simulink model "softloop1"  (Simulink 3.00)
settings: Solver=ode45  SolverMode=SingleTasking  StartTime=0.0  StopTime=25  MaxStep=.010  RelTol=1e-3  AbsTol=1e-3
settings Model: TimeSaveName=t  SaveOutput=off

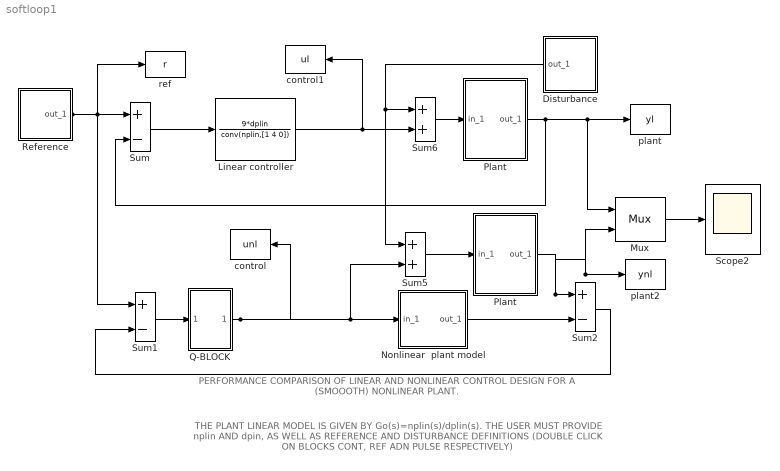
== system softloop1 ==
  note: THE PLANT LINEAR MODEL IS GIVEN BY Go(s)=nplin(s)/dplin(s).
      | THE USER MUST PROVIDE nplin AND dpin, AS WELL AS REFERENCE AND DISTURBANCE DEFINITIONS
      |  (DOUBLE CLICK ON BLOCKS CONT, REF ADN PULSE RESPECTIVELY)
  note: PERFORMANCE COMPARISON OF LINEAR AND NONLINEAR CONTROL DESIGN  FOR A
      | (SMOOOTH) NONLINEAR PLANT.
  Disturbance : Subsystem  Orientation=left  mask(Pulse disturbance){@1=0, @2=5, @3=10}
      mask prompts: @1 "pulse amplitude:"; @2 "initial time:"; @3 "pulse duration:"
      mask help: Pulse
      mask init:
      | D=@1;ti=@2;dt=@3;
      mask Help: This block generates a (one shot) pulse
      mask Display: disp('PULSE')
  Linear controller : TransferFcn  Numerator=9*dplin  Denominator=conv(nplin,[1 4 0])  mask(Controller){@1=1.13, @2=[1 3 1.55]}
      mask prompts: @1 "plant model numerator nplin:"; @2 "plant model denominator dplin:"
      mask help: Plant linear model
      mask init:
      | nplin=@1;dplin=@2;
      mask Display: disp('CONT')
  Mux : Mux  Inputs=2
      settings: DisplayOption=none
  "Nonlinear  plant model " : Subsystem
      mask Type: N.L.Model
      mask Display: disp('N.L.Mod')
  Plant : Subsystem
      mask Type: Plant
      mask Display: disp('Plant');
  "Plant " : Subsystem
      mask Type: Plant
      mask Display: disp('Plant')
  Q-BLOCK : Subsystem
  Reference : Subsystem  mask(Reference){@1=2, @2=0.3, @3=1}
      mask prompts: @1 "mean value Ro:"; @2 "square wave frequency   fsw  [rad/s]:"; @3 "amplitude square wave  asw:"
      mask help: Reference
      mask init:
      | Ro=@1;fsw=@2;asw=@3;
      mask Help: This block generates  a square wave with a user defined mean value.
      mask Display: disp('REF')
  Scope2 : Scope
      settings: TickLabels=on  TimeRange=25.000000  YMin=-4  YMax=4  SaveToWorkspace=off  SaveName=ScopeData  DataFormat=Matrix
  Sum : Sum  Inputs=+-  SaturateOnIntegerOverflow=on
  Sum1 : Sum  Inputs=+-  SaturateOnIntegerOverflow=on
  Sum2 : Sum  Inputs=+-  SaturateOnIntegerOverflow=on
  Sum5 : Sum  Inputs=++  SaturateOnIntegerOverflow=on
  Sum6 : Sum  Inputs=++  SaturateOnIntegerOverflow=on
  control : ToWorkspace  VariableName=unl  SampleTime=0  SaveFormat=Matrix
      settings: Buffer=10000
  control1 : ToWorkspace  VariableName=ul  SampleTime=0  SaveFormat=Matrix
      settings: Buffer=10000
  plant : ToWorkspace  VariableName=yl  SampleTime=0  SaveFormat=Matrix
      settings: Buffer=20000
  plant2 : ToWorkspace  VariableName=ynl  SampleTime=0  SaveFormat=Matrix
      settings: Buffer=20000
  ref : ToWorkspace  VariableName=r  SampleTime=0  SaveFormat=Matrix
      settings: Buffer=20000
  wires:
  Sum/1 -> Linear controller/1
  Plant/1(out_1) -> Sum/2, plant/1, Mux/1
  "Nonlinear  plant model "/1(out_1) -> Sum2/2
  Sum1/1 -> Q-BLOCK/1(in_1)
  Sum2/1 -> Sum1/2
  Q-BLOCK/1(out_1) -> control/1, "Nonlinear  plant model "/1(in_1), Sum5/2
  Sum5/1 -> "Plant "/1(in_1)
  "Plant "/1(out_1) -> Sum2/1, plant2/1, Mux/2
  Mux/1 -> Scope2/1
  Reference/1(out_1) -> Sum/1, Sum1/1, ref/1
  Sum6/1 -> Plant/1(in_1)
  Disturbance/1(out_1) -> Sum6/1, Sum5/1
  Linear controller/1 -> Sum6/2, control1/1

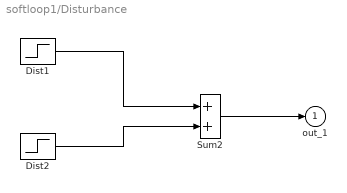
== system softloop1/Disturbance ==
  Dist1 : Step  Time=ti  Before=0  After=D  SampleTime=0
  Dist2 : Step  Time=ti+dt  Before=0  After=-D  SampleTime=0
  Sum2 : Sum  Inputs=++  SaturateOnIntegerOverflow=on
  out_1 : Outport  Port=1  InitialOutput=0
  wires:
  Sum2/1 -> out_1/1
  Dist1/1 -> Sum2/1
  Dist2/1 -> Sum2/2

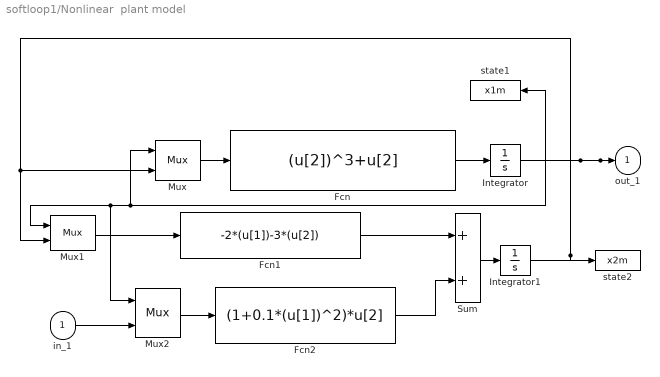
== system softloop1/Nonlinear  plant model  ==
  in_1 : Inport  Port=1  PortWidth=-1  SampleTime=-1  DataType=auto
      settings: SignalType=auto
  Fcn : Fcn  Expr=(u[2])^3+u[2]
  Fcn1 : Fcn  Expr=-2*(u[1])-3*(u[2])
  Fcn2 : Fcn  Expr=(1+0.1*(u[1])^2)*u[2]
  Integrator : Integrator  ExternalReset=none  InitialConditionSource=internal  InitialCondition=0  LimitOutput=off  UpperSaturationLimit=inf  LowerSaturationLimit=-inf  ShowSaturationPort=off  ShowStatePort=off  AbsoluteTolerance=auto
  Integrator1 : Integrator  ExternalReset=none  InitialConditionSource=internal  InitialCondition=0  LimitOutput=off  UpperSaturationLimit=inf  LowerSaturationLimit=-inf  ShowSaturationPort=off  ShowStatePort=off  AbsoluteTolerance=auto
  Mux : Mux  Inputs=2
      settings: DisplayOption=none
  Mux1 : Mux  Inputs=2
      settings: DisplayOption=none
  Mux2 : Mux  Inputs=2
      settings: DisplayOption=none
  Sum : Sum  Inputs=++  SaturateOnIntegerOverflow=on
  state1 : ToWorkspace  VariableName=x1m  SampleTime=0  SaveFormat=Matrix
      settings: Buffer=10000
  state2 : ToWorkspace  VariableName=x2m  SampleTime=0  SaveFormat=Matrix
      settings: Buffer=10000
  out_1 : Outport  Port=1  InitialOutput=0
  wires:
  in_1/1 -> Mux2/2
  Mux/1 -> Fcn/1
  Fcn/1 -> Integrator/1
  Mux1/1 -> Fcn1/1
  Fcn1/1 -> Sum/1
  Sum/1 -> Integrator1/1
  Fcn2/1 -> Sum/2
  Mux2/1 -> Fcn2/1
  Integrator/1 -> out_1/1, Mux/1, Mux1/1, Mux2/1, state1/1
  Integrator1/1 -> Mux1/2, Mux/2, state2/1

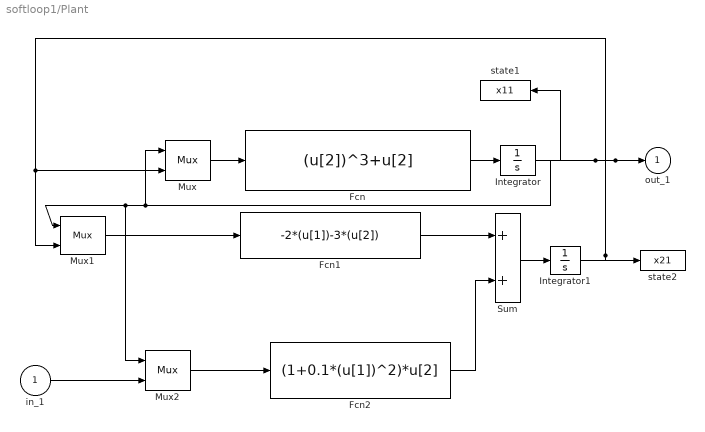
== system softloop1/Plant ==
  in_1 : Inport  Port=1  PortWidth=-1  SampleTime=-1  DataType=auto
      settings: SignalType=auto
  Fcn : Fcn  Expr=(u[2])^3+u[2]
  Fcn1 : Fcn  Expr=-2*(u[1])-3*(u[2])
  Fcn2 : Fcn  Expr=(1+0.1*(u[1])^2)*u[2]
  Integrator : Integrator  ExternalReset=none  InitialConditionSource=internal  InitialCondition=0  LimitOutput=off  UpperSaturationLimit=inf  LowerSaturationLimit=-inf  ShowSaturationPort=off  ShowStatePort=off  AbsoluteTolerance=auto
  Integrator1 : Integrator  ExternalReset=none  InitialConditionSource=internal  InitialCondition=0  LimitOutput=off  UpperSaturationLimit=inf  LowerSaturationLimit=-inf  ShowSaturationPort=off  ShowStatePort=off  AbsoluteTolerance=auto
  Mux : Mux  Inputs=2
      settings: DisplayOption=none
  Mux1 : Mux  Inputs=2
      settings: DisplayOption=none
  Mux2 : Mux  Inputs=2
      settings: DisplayOption=none
  Sum : Sum  Inputs=++  SaturateOnIntegerOverflow=on
  state1 : ToWorkspace  VariableName=x11  SampleTime=0  SaveFormat=Matrix
      settings: Buffer=10000
  state2 : ToWorkspace  VariableName=x21  SampleTime=0  SaveFormat=Matrix
      settings: Buffer=10000
  out_1 : Outport  Port=1  InitialOutput=0
  wires:
  in_1/1 -> Mux2/2
  Mux/1 -> Fcn/1
  Fcn/1 -> Integrator/1
  Mux1/1 -> Fcn1/1
  Fcn1/1 -> Sum/1
  Sum/1 -> Integrator1/1
  Fcn2/1 -> Sum/2
  Mux2/1 -> Fcn2/1
  Integrator/1 -> out_1/1, Mux/1, Mux1/1, Mux2/1, state1/1
  Integrator1/1 -> Mux1/2, Mux/2, state2/1

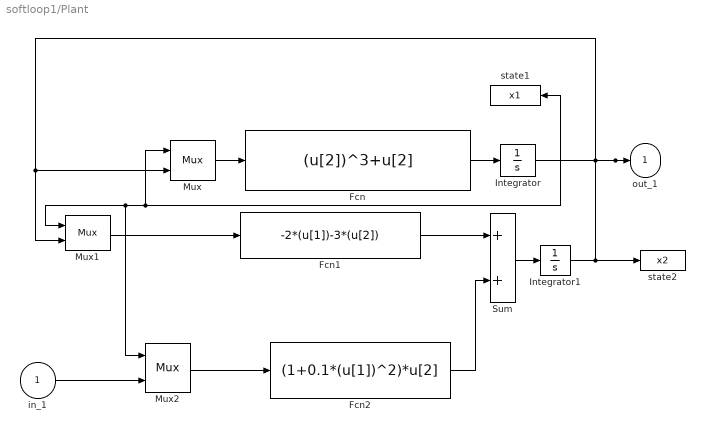
== system softloop1/Plant  ==
  in_1 : Inport  Port=1  PortWidth=-1  SampleTime=-1  DataType=auto
      settings: SignalType=auto
  Fcn : Fcn  Expr=(u[2])^3+u[2]
  Fcn1 : Fcn  Expr=-2*(u[1])-3*(u[2])
  Fcn2 : Fcn  Expr=(1+0.1*(u[1])^2)*u[2]
  Integrator : Integrator  ExternalReset=none  InitialConditionSource=internal  InitialCondition=0  LimitOutput=off  UpperSaturationLimit=inf  LowerSaturationLimit=-inf  ShowSaturationPort=off  ShowStatePort=off  AbsoluteTolerance=auto
  Integrator1 : Integrator  ExternalReset=none  InitialConditionSource=internal  InitialCondition=0  LimitOutput=off  UpperSaturationLimit=inf  LowerSaturationLimit=-inf  ShowSaturationPort=off  ShowStatePort=off  AbsoluteTolerance=auto
  Mux : Mux  Inputs=2
      settings: DisplayOption=none
  Mux1 : Mux  Inputs=2
      settings: DisplayOption=none
  Mux2 : Mux  Inputs=2
      settings: DisplayOption=none
  Sum : Sum  Inputs=++  SaturateOnIntegerOverflow=on
  state1 : ToWorkspace  VariableName=x1  SampleTime=0  SaveFormat=Matrix
      settings: Buffer=10000
  state2 : ToWorkspace  VariableName=x2  SampleTime=0  SaveFormat=Matrix
      settings: Buffer=10000
  out_1 : Outport  Port=1  InitialOutput=0
  wires:
  in_1/1 -> Mux2/2
  Mux/1 -> Fcn/1
  Fcn/1 -> Integrator/1
  Mux1/1 -> Fcn1/1
  Fcn1/1 -> Sum/1
  Sum/1 -> Integrator1/1
  Fcn2/1 -> Sum/2
  Mux2/1 -> Fcn2/1
  Integrator/1 -> out_1/1, Mux/1, Mux1/1, Mux2/1, state1/1
  Integrator1/1 -> Mux1/2, Mux/2, state2/1

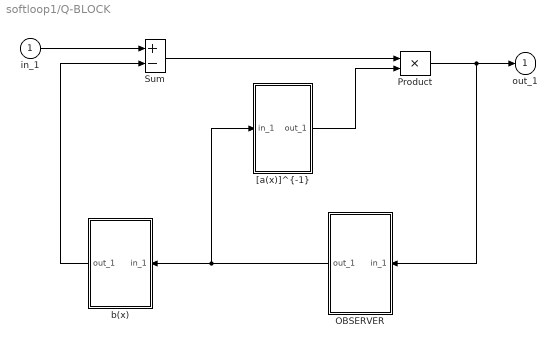
== system softloop1/Q-BLOCK ==
  in_1 : Inport  Port=1  PortWidth=-1  SampleTime=-1  DataType=auto
      settings: SignalType=auto
  OBSERVER : Subsystem  Orientation=left
  Product : Product  Inputs=2  SaturateOnIntegerOverflow=on
  Sum : Sum  Inputs=+-  SaturateOnIntegerOverflow=on
  "[a(x)]^{-1}" : Subsystem
  b(x) : Subsystem  Orientation=left
  out_1 : Outport  Port=1  InitialOutput=0
  wires:
  OBSERVER/1(out_1) -> b(x)/1(in_1), "[a(x)]^{-1}"/1(in_1)
  Product/1 -> out_1/1, OBSERVER/1(in_1)
  "[a(x)]^{-1}"/1(out_1) -> Product/2
  b(x)/1(out_1) -> Sum/2
  Sum/1 -> Product/1
  in_1/1 -> Sum/1

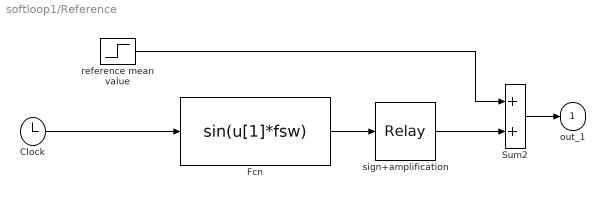
== system softloop1/Reference ==
  Clock : Clock
      settings: DisplayTime=off  Decimation=10
  Fcn : Fcn  Expr=sin(u[1]*fsw)
  Sum2 : Sum  Inputs=++  SaturateOnIntegerOverflow=on
  reference mean value : Step  Time=0  Before=0  After=Ro  SampleTime=0
  sign+amplification : Relay  OnSwitchValue=0  OffSwitchValue=0  OnOutputValue=asw  OffOutputValue=-asw
  out_1 : Outport  Port=1  InitialOutput=0
  wires:
  sign+amplification/1 -> Sum2/2
  Fcn/1 -> sign+amplification/1
  Clock/1 -> Fcn/1
  Sum2/1 -> out_1/1
  reference mean value/1 -> Sum2/1

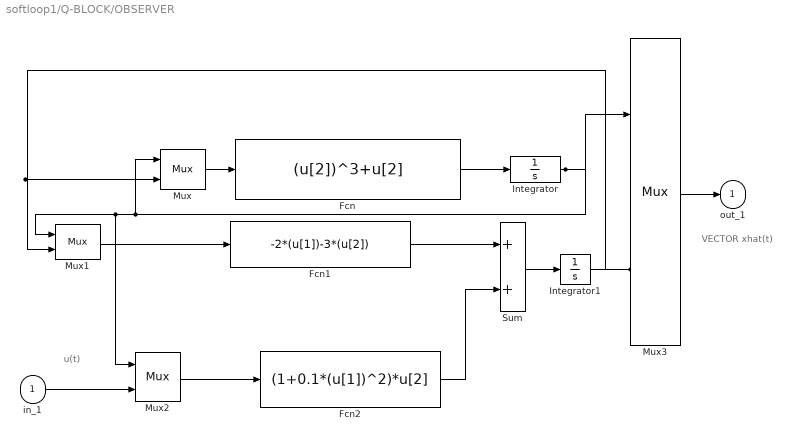
== system softloop1/Q-BLOCK/OBSERVER ==
  note: u(t)
  note: VECTOR
      |   xhat(t)
  in_1 : Inport  Port=1  PortWidth=-1  SampleTime=-1  DataType=auto
      settings: SignalType=auto
  Fcn : Fcn  Expr=(u[2])^3+u[2]
  Fcn1 : Fcn  Expr=-2*(u[1])-3*(u[2])
  Fcn2 : Fcn  Expr=(1+0.1*(u[1])^2)*u[2]
  Integrator : Integrator  ExternalReset=none  InitialConditionSource=internal  InitialCondition=0  LimitOutput=off  UpperSaturationLimit=inf  LowerSaturationLimit=-inf  ShowSaturationPort=off  ShowStatePort=off  AbsoluteTolerance=auto
  Integrator1 : Integrator  ExternalReset=none  InitialConditionSource=internal  InitialCondition=0  LimitOutput=off  UpperSaturationLimit=inf  LowerSaturationLimit=-inf  ShowSaturationPort=off  ShowStatePort=off  AbsoluteTolerance=auto
  Mux{,1..3} (4 alike) : Mux  Inputs=2
      settings: DisplayOption=none
  Sum : Sum  Inputs=++  SaturateOnIntegerOverflow=on
  out_1 : Outport  Port=1  InitialOutput=0
  wires:
  Mux2/1 -> Fcn2/1
  Fcn2/1 -> Sum/2
  Sum/1 -> Integrator1/1
  Fcn1/1 -> Sum/1
  Mux1/1 -> Fcn1/1
  Fcn/1 -> Integrator/1
  Mux/1 -> Fcn/1
  Integrator/1 -> Mux1/1, Mux2/1, Mux/1, Mux3/1
  in_1/1 -> Mux2/2
  Mux3/1 -> out_1/1
  Integrator1/1 -> Mux3/2, Mux1/2, Mux/2

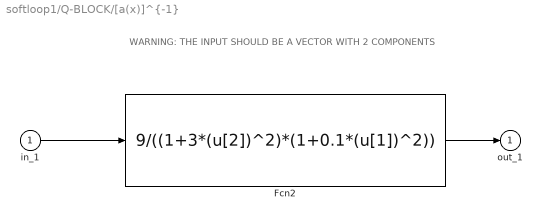
== system softloop1/Q-BLOCK/[a(x)]^{-1} ==
  note: WARNING: THE INPUT SHOULD BE A VECTOR WITH 2 COMPONENTS
  in_1 : Inport  Port=1  PortWidth=-1  SampleTime=-1  DataType=auto
      settings: SignalType=auto
  Fcn2 : Fcn  Expr=9/((1+3*(u[2])^2)*(1+0.1*(u[1])^2))
  out_1 : Outport  Port=1  InitialOutput=0
  wires:
  in_1/1 -> Fcn2/1
  Fcn2/1 -> out_1/1

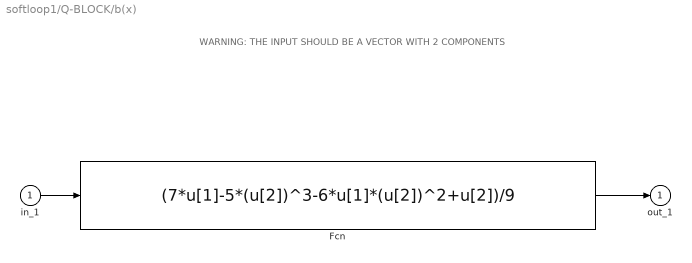
== system softloop1/Q-BLOCK/b(x) ==
  note: WARNING: THE INPUT SHOULD BE A VECTOR WITH 2 COMPONENTS
  in_1 : Inport  Port=1  PortWidth=-1  SampleTime=-1  DataType=auto
      settings: SignalType=auto
  Fcn : Fcn  Expr=(7*u[1]-5*(u[2])^3-6*u[1]*(u[2])^2+u[2])/9
  out_1 : Outport  Port=1  InitialOutput=0
  wires:
  in_1/1 -> Fcn/1
  Fcn/1 -> out_1/1
